simulink library "ESTS_TFY_LatAxle"  (R2022a)
settings: Solver=VariableStepAuto  StartTime=0.0  StopTime=10.0  RelTol=1e-3
undefined symbols (not defined in the file): p_JzVeh_kgm2
libraries: VUT_lib x1
settings Model: Creator=blatak  LastModifiedBy=blatak

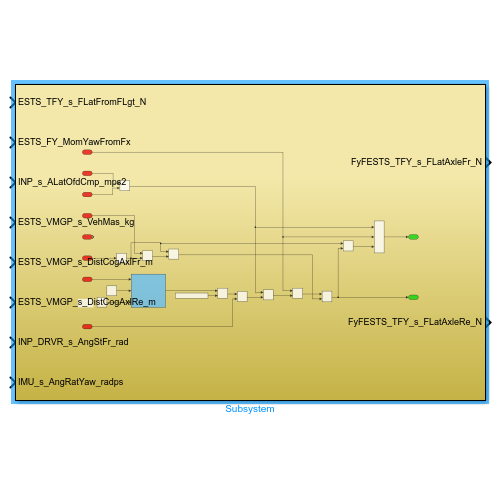
[thumbnail: Simulink's stored preview of the top-level diagram]
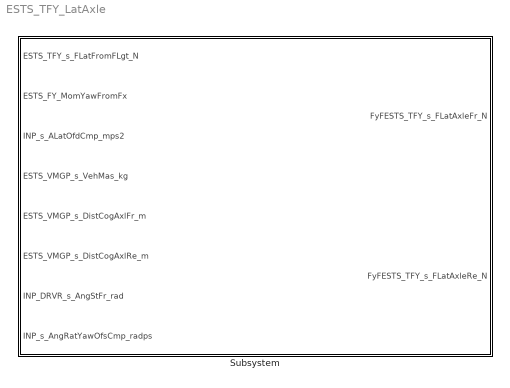
== system ESTS_TFY_LatAxle ==
  Subsystem : Subsystem

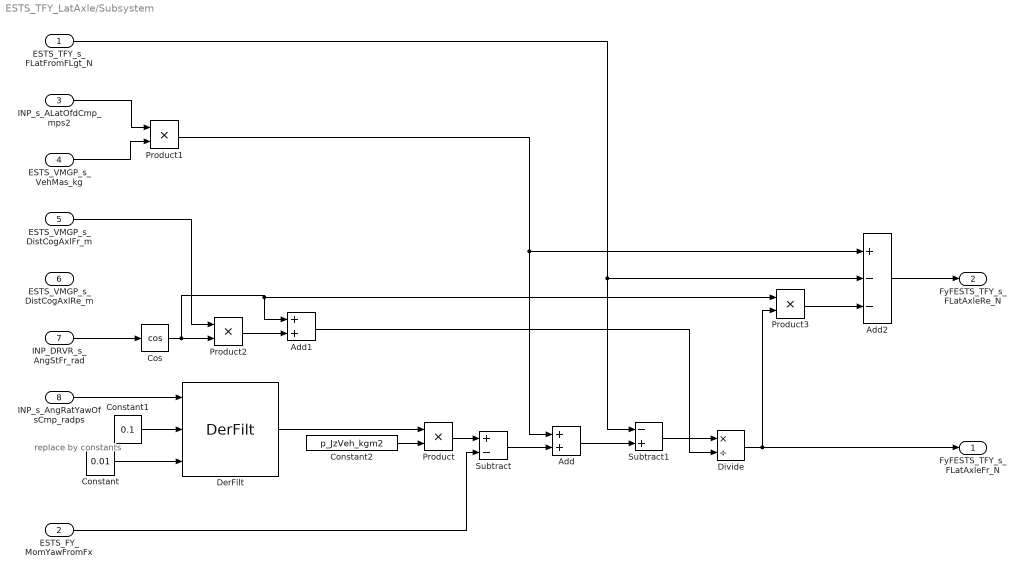
== system ESTS_TFY_LatAxle/Subsystem ==
  note: replace by
      | constants
  ESTS_TFY_s_FLatFromFLgt_N : Inport
  ESTS_FY_MomYawFromFx : Inport  Port=2
  INP_s_ALatOfdCmp_mps2 : Inport  Port=3
  ESTS_VMGP_s_VehMas_kg : Inport  Port=4
  ESTS_VMGP_s_DistCogAxlFr_m : Inport  Port=5
  ESTS_VMGP_s_DistCogAxlRe_m : Inport  Port=6
  INP_DRVR_s_AngStFr_rad : Inport  Port=7
  INP_s_AngRatYawOfsCmp_radps : Inport  Port=8
  Add : Sum
  Add1 : Sum
  Add2 : Sum  Inputs=+--
  Constant : Constant  Value=0.01  OutDataTypeStr=single
  Constant1 : Constant  Value=0.1  OutDataTypeStr=single
  Constant2 : Constant  Value=p_JzVeh_kgm2
  Cos : Trigonometry  Operator=cos
  DerFilt : VUT_lib/DerFilt  SystemSampleTime=-1  VariantActivationTime=update diagram  Latency=0  AutoFrameSizeCalculation=off
  Divide : Product  Inputs=*/  RndMeth=Zero  SaturateOnIntegerOverflow=on
  Product{,1..3} (4 alike) : Product
  Subtract : Sum  Inputs=+-
  Subtract1 : Sum  Inputs=-+
  FyFESTS_TFY_s_FLatAxleFr_N : Outport
  FyFESTS_TFY_s_FLatAxleRe_N : Outport  Port=2
  wires:
  INP_s_AngRatYawOfsCmp_radps/1 -> DerFilt/1
  Constant/1 -> DerFilt/3
  Constant1/1 -> DerFilt/2
  DerFilt/1 -> Product/1
  Constant2/1 -> Product/2
  ESTS_FY_MomYawFromFx/1 -> Subtract/2
  INP_s_ALatOfdCmp_mps2/1 -> Product1/1
  ESTS_VMGP_s_VehMas_kg/1 -> Product1/2
  Product/1 -> Subtract/1
  Subtract/1 -> Add/2
  Product1/1 -> Add2/1, Add/1
  Add/1 -> Subtract1/2
  ESTS_TFY_s_FLatFromFLgt_N/1 -> Add2/2, Subtract1/1
  INP_DRVR_s_AngStFr_rad/1 -> Cos/1
  Cos/1 -> Add1/1, Product3/1, Product2/2
  ESTS_VMGP_s_DistCogAxlFr_m/1 -> Product2/1
  Product2/1 -> Add1/2
  Subtract1/1 -> Divide/1
  Add1/1 -> Divide/2
  Divide/1 -> Product3/2, FyFESTS_TFY_s_FLatAxleFr_N/1
  Product3/1 -> Add2/3
  Add2/1 -> FyFESTS_TFY_s_FLatAxleRe_N/1
